simulink model "Distribute2a_Model"  (R2023a)
settings: Solver=VariableStepAuto  StartTime=0.0  StopTime=10.0  RelTol=1e-3
libraries: NSA_DEVS_LOGISTICS_ATOMIC x4, NSA_DEVS_SINKS_ATOMIC x3, NSA_DEVS_ROUTING_ATOMIC x1, NSA_DEVS_SOURCES_ATOMIC x1
settings Model: Creator=david  LastModifiedBy=peter

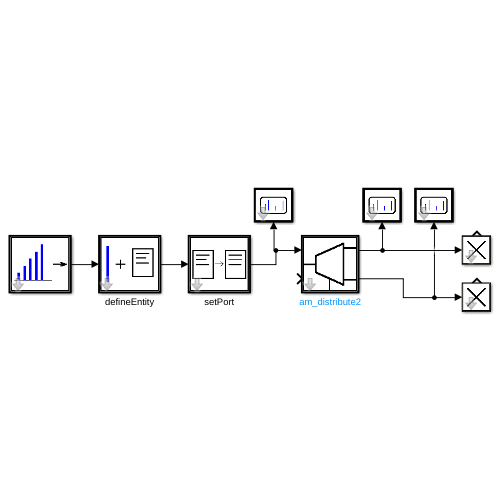
[thumbnail: Simulink's stored preview of the top-level diagram]
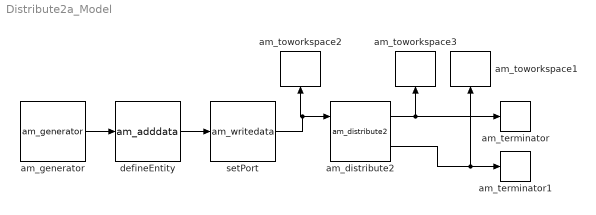
== system Distribute2a_Model ==
  am_distribute2 : NSA_DEVS_ROUTING_ATOMIC/am_distribute2  port0=1  field="\"port\""  tau=[0,1]  debug=0
      settings: SourceProductName=NSA_DEVS
  am_generator : NSA_DEVS_SOURCES_ATOMIC/am_generator  tG=1  n0=1  nG=9  tD=[0,2]  debug=0
      settings: SourceProductName=NSA_DEVS
  am_terminator : NSA_DEVS_LOGISTICS_ATOMIC/am_terminator  tau=[0,1]  debug=0
      settings: SourceProductName=NSA_DEVS
  am_terminator1 : NSA_DEVS_LOGISTICS_ATOMIC/am_terminator  tau=[0,1]  debug=0
      settings: SourceProductName=NSA_DEVS
  am_toworkspace1 : NSA_DEVS_SINKS_ATOMIC/am_toworkspace  varname="\"dataOut2\""  t0=0  format="\"vector\""  tau=[0,3]  debug=0
      settings: SourceProductName=NSA_DEVS
  am_toworkspace2 : NSA_DEVS_SINKS_ATOMIC/am_toworkspace  varname="\"dataIn\""  t0=0  format="\"vector\""  tau=[0,3]  debug=0
      settings: SourceProductName=NSA_DEVS
  am_toworkspace3 : NSA_DEVS_SINKS_ATOMIC/am_toworkspace  varname="\"dataOut1\""  t0=0  format="\"vector\""  tau=[0,3]  debug=0
      settings: SourceProductName=NSA_DEVS
  defineEntity : NSA_DEVS_LOGISTICS_ATOMIC/am_adddata  fields="[\"port\"]"  values="[\"1\"]"  numeric=[true]  infield="\"id\""  tau=[0,1]  debug=0
      settings: SourceProductName=NSA_DEVS
  setPort : NSA_DEVS_LOGISTICS_ATOMIC/am_writedata  inFields=[]  outField="\"port\""  changeFunc="\"out = randi(2);\""  tau=[0,1]  debug=0
      settings: SourceProductName=NSA_DEVS
  wires:
  am_generator/1 -> defineEntity/1
  defineEntity/1 -> setPort/1
  am_distribute2/1 -> am_terminator/1, am_toworkspace3/1
  setPort/1 -> am_distribute2/1, am_toworkspace2/1
  am_distribute2/2 -> am_terminator1/1, am_toworkspace1/1
